simulink model "OFDM_model_v2020"  (R2020b)
settings: Solver=FixedStepDiscrete  StartTime=0.0  StopTime=inf  RelTol=1e-3
PreLoadFcn:
  | % [(TsOFDM/64)/1e3 (TsOFDM/64)/1e2]
InitFcn:
  | %%% SELECTIONNEZ LES PARAMETRES DU MODELE %%%
  | 
  | Te = 30e-9; % temps entre deux échantillons au niveau du canal
  | N = 219; % nombre total de sous-porteuses
  | pilots_inter = 2; % nombre de sous-canaux entre deux pilotes
  | prefix_len = 26; % taille du préfixe cyclique
  | 
  | path_delays = [Te 10*Te];
  | path_gains = [-3 -6];
  | 
  | 
  | 
  | %%% NE PAS MODIFIER %%%
  | 
  | pilots_per_sym = 128/2+1 % nombre de pilotes par symbole OFDM  (N - prefix_len + pilots_inter)/(pilots_inter+1);
  | 
  | N_data = N - prefix_len - pilots_per_sym;
  | 
  | TsOFDM = N*Te; % temps symbole
  | 
  | 
  | 
  | %%% VERIFICATION DES CONDITIONS SUR LES PARAMETRES %%%
  | 
  | if N/Te >= 20e6 %
  |     %error('La bande doit être inférieure à 20Mhz. Augmentez Te ou diminuez N.');
  | end
  | 
  | if TsOFDM <= max(path_delays)
  |     %error('Le fading doit être plat dans chaque sous-canal. Augmentez Te ou diminuez le delai max.');
  | end
  | 
  | if mod(pilots_per_sym, 1) ~= 0 || pilots_per_sym < 2
  |    % error('Un symbole OFDM doit contenir un nombre entier de pilotes. Modifiez N, pilots_inter ou prefix_len.');
  | end
  | 
  | for i = 1:length(path_delays)
  |     if mod( Te, path_delays(i) ) ~= 0
  |         %error('Les délais doivent être des multiples du sample time.');
  |     end
  | end
  | 
  | if 9*Te < max(path_delays)
  |     %error('Le temps de garde entre doit être supérieur ou égal au delai max. Augmentez prefix_length ou diminuez le delai max.');
  | end
  | 
  | 
  | 
  | 
  | 
  | 
  | 
  | 
  | 
  | 
  | % BsOFDM = 1/TsOFDM; % largeur de bande d'un symbole
  | 
  | % TgOFDM = 0.1*TsOFDM; % temps de garde
  | 
  | % A CHECK TcoOFDM = 6*TsOFDM; % temps de cohérence du canal
  | % A CHECK BcoOFDM = 1/TcoOFDM; % bande de cohérence du canal
  | 
  | % prefix_len = floor(TgOFDM/(TsOFDM/N)); % taille du préfixe cyclique
  | % refix_len = 5 ;
  | 
  | % sym_per_pilot = floor(TcoOFDM/TsOFDM) - 1; % nombre de symboles pendant lesquels le pilote est valable (méthode 1)
  | % channels_per_pilot = 4 % A CHECK floor(BcoOFDM/BsOFDM) - 1; % nombre de sous-canaux sur lesquels le pilote est valable (métohde 2)
  | 
  | % pilots_per_sym = int8( floor( N / channels_per_pilot ) ); % nombre de pilotes par symbole (préfixe comrpis)
undefined symbols (not defined in the file or in its folder): doppler
libraries: dspindex x3, dspxfrm3 x2, commdigbbndpm3 x2, commchan3 x2, commrandsrc3 x1, commsink2 x1, commutil2 x1
Description:
  | This model uses Universal Software Radio Peripheral (USRP) hardware with Simulink(R) to perform FM demodulation and stereo decoding.
settings Model: SimulationMode=accelerator  Creator=nicol  LastModifiedBy=nicol
settings DataIOCC: SaveFormat=Structure  SaveOutput=off  SignalLogging=off  DSMLogging=off  SaveTime=off  ReturnWorkspaceOutputs=off
settings OptimizationCC: ExpressionDepthLimit=2147483647  EfficientMapNaN2IntZero=off  LifeSpan=inf  SimCompilerOptimization=on
settings DebuggingCC: UnderspecifiedInitializationDetection=Classic  MergeDetectMultiDrivingBlocksExec=none  SolverPrmCheckMsg=warning  InheritedTsInSrcMsg=none  MultiTaskCondExecSysMsg=none  ParameterPrecisionLossMsg=none  FcnCallInpInsideContextMsg=warning  AllowSymbolicDim=off  StateNameClashWarn=warning  SFUnexpectedBacktrackingDiag=warning  SFNoUnconditionalDefaultTransitionDiag=warning  SFExecutionAtInitializationDiag=none  ArithmeticOperatorsInVariantConditions=warning
settings HardwareCC: ProdBitPerPointer=32  ProdBitPerSizeT=32  ProdBitPerPtrDiffT=32  ProdLargestAtomicFloat=None  ProdIntDivRoundTo=Undefined  ProdEndianess=Unspecified  ProdWordSize=32  ProdHWDeviceType=32-bit Generic  TargetBitPerPointer=64  TargetBitPerSizeT=64  TargetBitPerPtrDiffT=64  TargetLongLongMode=on  TargetIntDivRoundTo=Zero  TargetEndianess=LittleEndian  TargetWordSize=64  TargetHWDeviceType=Generic->MATLAB Host Computer  ProdEqTarget=off
settings ModelReferenceCC: PropagateSignalLabelsOutOfModel=off
settings SFSimCC: SimIntegrity=off  SimUseLocalCustomCode=off  CustomCodeUndefinedFunction=UseInterfaceOnly
settings RTWCC: RTWUseLocalCustomCode=off
settings RTWCC: CustomSourceCode=|
  | #include <stdio.h>
  | #include <stdlib.h>
settings CodeAppCC: MaxIdLength=128  StateflowObjectComments=on
settings GRTTargetCC: TargetLangStandard=C89/C90 (ANSI)  CombineOutputUpdateFcns=off  GRTInterface=on
settings ConfigComp: CovMetricSettings=dw  CovSaveCumulativeToWorkspaceVar=on  CovSaveSingleToWorkspaceVar=on  CovExternalEMLEnable=off  CovSFcnEnable=off

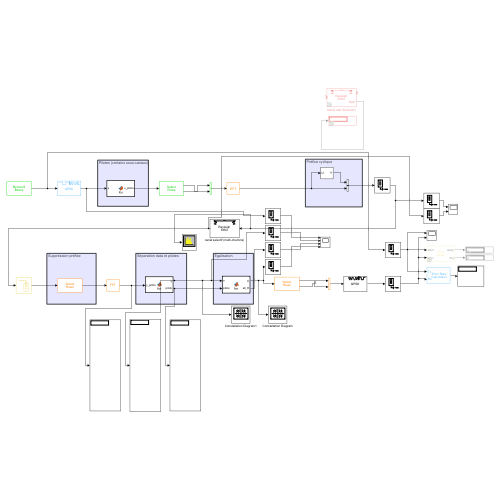
[thumbnail: Simulink's stored preview of the top-level diagram]
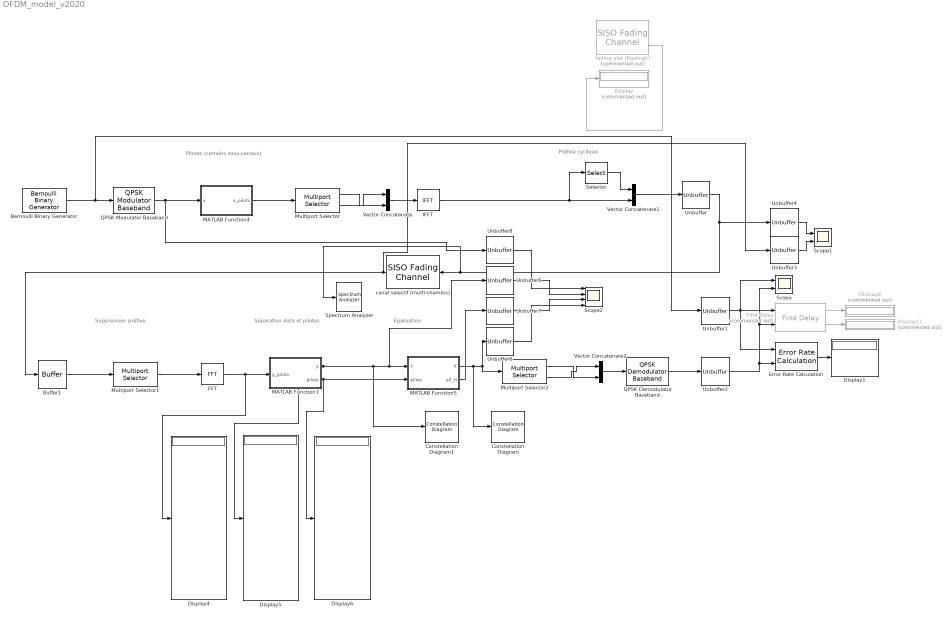
== system OFDM_model_v2020 ==
  note: Égalisation
  note: Séparation data et pilotes
  note: Suppression préfixe
  note: Préfixe cyclique
  note: Pilotes (certains sous-canaux)
  Bernoulli Binary Generator : commrandsrc3/Bernoulli Binary Generator  ProbabilityOfZero=0.5  SeedSource=Parameter  Seed=252  SampleTime=(N*Te)/(2*N_data)  SamplesPerFrame=2*N_data  OutputDataType=double  SimulateUsing=Code generation
  Buffer1 : Buffer  N=N  OutputFrames=off
  Constellation Diagram : ConstellationDiagram
  Constellation Diagram1 : ConstellationDiagram
  Display : Display  Commented=on
  Display{1,4..6} (4 alike) : Display
  Display11 : Display  Commented=on
  Display8 : Display  Commented=on
  Error Rate Calculation : commsink2/Error Rate Calculation  N=256  st_delay=0  cp_mode=Entire frame  subframe=[]  PMode=Port  WsName=ErrorVec  RsMode2=off  stop=off  numErr=100  maxBits=1e6
  FFT : dspxfrm3/FFT  FFTImplementation=Auto  CompMethod=Table lookup  TableOpt=NEW  TableOptActive=Speed  BitRevOrder=off  Normalize=off  InheritFFTLength=on  FFTLength=64  WrapInput=on  roundingMode=Floor  overflowMode=off  firstCoeffDataTypeStr=Inherit: Same word length as input  firstCoeffLastDataTypeStr=Inherit: Same word length as input  outputMin=[]  outputMax=[]
  Find Delay : commutil2/Find Delay  Commented=on  corrLength=500  chgSigOP=on  stopUpdate=off  numConstDelay=3
      settings: SourceProductBaseCode=CM
  IFFT : dspxfrm3/IFFT  FFTImplementation=Auto  CompMethod=Table lookup  TableOpt=NEW  TableOptActive=Speed  BitRevOrder=off  cs_in=off  Normalize=on  InheritFFTLength=on  FFTLength=64  WrapInput=on  mode=Complex  outSamplingMode=Sample based  roundingMode=Floor  overflowMode=off  firstCoeffDataTypeStr=Inherit: Same word length as input  firstCoeffLastDataTypeStr=Inherit: Same word length as input  outputMin=[]  outputMax=[]
  MATLAB Function1 : MATLAB Function  TreatAsAtomicUnit=on
  MATLAB Function4 : MATLAB Function  TreatAsAtomicUnit=on
  MATLAB Function5 : MATLAB Function  TreatAsAtomicUnit=on
  Multiport Selector : dspindex/Multiport Selector  rowsOrCols=Rows  idxCellArray={1 : 1+(N_data+pilots_per_sym)/2, (N_data+pilots_per_sym)/2+1 : N_data+pilots_per_sym}  idxErrMode=Clip Index
  Multiport Selector1 : dspindex/Multiport Selector  rowsOrCols=Rows  idxCellArray=[ prefix_len + 1 : N]  idxErrMode=Clip Index
  Multiport Selector2 : dspindex/Multiport Selector  rowsOrCols=Rows  idxCellArray={1 : N_data/2, N_data/2+1 : N_data}  idxErrMode=Clip Index
  QPSK Demodulator Baseband : commdigbbndpm3/QPSK Demodulator Baseband  OutType=Bit  DecType=Hard decision  VarSource=Dialog  Variance=1  Dec=Gray  Ph=pi/4  outDtype1=Inherit via internal rule  outDtype2=Inherit via internal rule  derotateFactorWordLen=16  derotateFactorDataTypeStr=Inherit: Same word length as input  derotateFactorLastDataTypeStr=Inherit: Same word length as input
  QPSK Modulator Baseband : commdigbbndpm3/QPSK Modulator Baseband  InType=Bit  Enc=Gray  Ph=pi/4  outDtype=double  outWordLen=16  outUDDataType=sfix(16)  outFracLenMode=Best precision  outFracLen=15  outDataTypeStr=double  outLastDataTypeStr=double
  Scope : Scope  NumInputPorts=2
  Scope1 : Scope  NumInputPorts=2
  Scope2 : Scope  NumInputPorts=4
  Selector : Selector  InputPortWidth=N_data + pilots_per_sym  IndexOptions=Index vector (dialog)  Indices=[N_data + pilots_per_sym - prefix_len + 1 : N_data + pilots_per_sym]  OutputSizes=1
  Spectrum Analyzer : SpectrumAnalyzer
  Unbuffer{,1..8} (9 alike) : Unbuffer
  Vector Concatenate : Concatenate
  Vector Concatenate1 : Concatenate
  Vector Concatenate2 : Concatenate
  canal selectif (multi-chemins) : commchan3/SISO Fading Channel  InheritSampleRate=on  SampleRate=1  PathDelays=path_delays  AveragePathGains=path_gains  NormalizePathGains=on  FadingDistribution=Rayleigh  KFactor=3  DirectPathDopplerShift=0  DirectPathInitialPhase=0  MaximumDopplerShift=100  DopplerSpectrum=doppler('Jakes')  RandomStream=mt19937ar with seed  Seed=73  PathGainsOutputPort=off  ChannelFilterDelayOutputPort=off  SimulateUsing=Code generation  Visualization=Off  PathsForDopplerDisplay=1  SamplesToDisplay=25%
  fading plat (Rayleigh) : commchan3/SISO Fading Channel  Commented=on  InheritSampleRate=on  SampleRate=1  PathDelays=0  AveragePathGains=0  NormalizePathGains=on  FadingDistribution=Rayleigh  KFactor=3  DirectPathDopplerShift=0  DirectPathInitialPhase=0  MaximumDopplerShift=20  DopplerSpectrum=doppler('Jakes')  RandomStream=mt19937ar with seed  Seed=73  PathGainsOutputPort=on  ChannelFilterDelayOutputPort=off  SimulateUsing=Code generation  Visualization=Off  PathsForDopplerDisplay=1  SamplesToDisplay=25%
  wires:
  Bernoulli Binary Generator/1 -> QPSK Modulator Baseband/1, Unbuffer1/1
  QPSK Modulator Baseband/1 -> Unbuffer8/1, MATLAB Function4/1(x)
  Multiport Selector/2 -> Vector Concatenate/1
  Multiport Selector/1 -> Vector Concatenate/2
  Vector Concatenate/1 -> IFFT/1
  fading plat (Rayleigh)/2 -> Display/1
  canal selectif (multi-chemins)/1 -> Unbuffer3/1, Buffer1/1
  Error Rate Calculation/1 -> Display1/1
  Selector/1 -> Vector Concatenate1/1
  Find Delay/1 -> Display8/1
  Find Delay/2 -> Display11/1
  IFFT/1 -> Selector/1, Vector Concatenate1/2
  MATLAB Function1/1(y) -> Display5/1, Constellation Diagram1/1, MATLAB Function5/1(Y), Unbuffer5/1
  MATLAB Function1/2(pilots) -> Display6/1, MATLAB Function5/2(pilots)
  Unbuffer2/1 -> Scope/2, Find Delay/2, Error Rate Calculation/2
  Unbuffer1/1 -> Error Rate Calculation/1, Scope/1, Find Delay/1
  QPSK Demodulator Baseband/1 -> Unbuffer2/1
  MATLAB Function5/1(X) -> Constellation Diagram/1, Multiport Selector2/1, Unbuffer6/1
  Multiport Selector2/1 -> Vector Concatenate2/2
  Multiport Selector2/2 -> Vector Concatenate2/1
  Vector Concatenate2/1 -> QPSK Demodulator Baseband/1
  Vector Concatenate1/1 -> Unbuffer/1
  Unbuffer/1 -> Unbuffer4/1, Spectrum Analyzer/1, canal selectif (multi-chemins)/1
  Buffer1/1 -> Multiport Selector1/1
  Unbuffer5/1 -> Scope2/2
  Unbuffer6/1 -> Scope2/4
  MATLAB Function5/2(all_H) -> Unbuffer7/1
  Unbuffer7/1 -> Scope2/3
  Unbuffer8/1 -> Scope2/1
  Unbuffer4/1 -> Scope1/1
  Unbuffer3/1 -> Scope1/2
  MATLAB Function4/1(x_pilots) -> Multiport Selector/1
  Multiport Selector1/1 -> FFT/1
  FFT/1 -> MATLAB Function1/1(y_pilots), Display4/1

== matlab function OFDM_model_v2020/MATLAB Function1 ==
  data: y_pilots input; y output; pilots output; pilots_inter parameter; pilots_per_sym parameter; N_data parameter
function [y, pilots] = fcn(y_pilots, pilots_inter, pilots_per_sym, N_data)

pilots = complex(0, 0) * ones(pilots_per_sym, 1);
y = complex(0, 0) * ones(N_data, 1);

p_counter = 1;
s_counter = 1;

for idx = 1:length(y_pilots)
    if mod(idx-1, pilots_inter+1) ~= 0
        y(s_counter) = y_pilots(idx);
        s_counter = s_counter + 1;
    else
       pilots(p_counter) = y_pilots(idx);
       p_counter = p_counter + 1;
    end
end



%{
pilots = in(1:channels_per_pilot+2:length(in)); % vecteur contenant tous les pilotes du symbole

dup_pilots_bis = complex((1:30), (1:30));
dup_pilots_bis(1) = pilots(1);

for i = 2:length(pilots)-1
    dup_pilots_bis(2*(i-2)+2) = pilots(i);
    dup_pilots_bis(2*(i-2)+2+1) = pilots(i);
end

dup_pilots_bis(end) = pilots(end);

dup_pilots = dup_pilots_bis';


Y = in(setdiff(1:length(i), 1:channels_per_pilot+1:length(i))); % vecteur contenant tous les échantillons du symbole      
%}

== matlab function OFDM_model_v2020/MATLAB Function4 ==
  data: x input; x_pilots output; pilots_inter parameter; pilots_per_sym parameter; N_data parameter
function x_pilots = fcn(x, pilots_inter, pilots_per_sym, N_data)

x_pilots = complex(0, 0) * ones(N_data + pilots_per_sym, 1); % symbole OFDM avec pilotes

s_counter = 1; % variable d'itération sur X (symbole OFDM s sans pilotes)

for idx = 1:length(x_pilots)
    if mod(idx-1, pilots_inter+1) ~= 0
        x_pilots(idx) = x(s_counter);
        s_counter = s_counter + 1;
    else
        x_pilots(idx) = 10+10i;
    end
end

== matlab function OFDM_model_v2020/MATLAB Function5 ==
  data: Y input; X output; pilots input; pilots_per_sym parameter; N_data parameter; pilots_inter parameter; all_H output
function [X,all_H] = fcn(Y, pilots, pilots_per_sym, N_data, pilots_inter)

%ReY = real(Y);
%ImY = imag(Y);

X = complex(0, 0) * ones(N_data, 1);
all_H = complex(0, 0) * ones(N_data, 1); %tmp


for bloc_idx = 0:pilots_per_sym-2
    left_pilot = pilots(bloc_idx+1);
    right_pilot = pilots(bloc_idx+2);

    %left_H = complex(real(left_pilot)/10, imag(left_pilot)/10);
    %right_H = complex(real(right_pilot)/10, imag(right_pilot)/10);

    left_H = left_pilot/(10+10i);
    right_H = right_pilot/(10+10i);

    pilots_interp = linspace(left_H, right_H, pilots_inter + 2);

    H_interp = pilots_interp(2:end-1);

    %ReH = real(H_interp);
    %ImH = imag(H_interp);

   for sample = 1:pilots_inter
       %ReY_s = ReY(pilots_inter*bloc_idx+sample);
       %ImY_s = ImY(pilots_inter*bloc_idx+sample);
       Y_s = Y(pilots_inter*bloc_idx+sample);

       %X(pilots_inter*bloc_idx+sample) = complex( ReY_s./ReH(sample), ImY_s./ImH(sample) );
       X(pilots_inter*bloc_idx+sample) = Y_s/H_interp(sample);
       %all_H(pilots_inter*bloc_idx+sample) = complex(ReH(sample), ImH(sample));
       all_H(pilots_inter*bloc_idx+sample) = H_interp(sample);
   end

end
